simulink model "Lidar_System_July7_NoSerial"  (Simulink 7.3)
settings: Solver=FixedStepDiscrete  StartTime=0.0  StopTime=inf  FixedStep=0.1  MaxStep=0.2  RelTol=1e-3
libraries: dspmtrx3 x3, simulink x2, vipstatistics x2, dspstat3 x2, vipgeotforms x1
(part 1 of 2)
settings Model: Creator=gclayton  LastModifiedBy=wildcat
settings DebuggingCC: InheritedTsInSrcMsg=none
settings RTWCC: SystemTargetFile=rlnx.tlc  GenCodeOnly=on  TemplateMakefile=rlnx_ubuntu.tmf  Description=Linux Real-Time Target  ProcessScript=rlnx_make_rtw_hook
settings RTWCC: CustomInclude=|
  | /usr/local/include/opencv/
  | /usr/local/include/
settings CodeAppCC: GenerateComments=off  SimulinkBlockComments=off
settings STFCustomTargetCC: ModelReferenceCompliant=off  MatFileLogging=on  SystemTargetFile=rlnx.tlc
settings GRTTargetCC: ModelReferenceCompliant=off  ParMdlRefBuildCompliant=off  CompOptLevelCompliant=off
settings CustomProperty: DataType=string  Value="-lm -ldl /usr/local/lib/libopencv_highgui.so.2.4 /usr/local/lib/libopencv_core.so.2.4 /usr/local/lib/libopencv_imgproc.so.2.4  -lc_urg -lc_urg_connection -lc_urg_system -lphidget21"
settings EnumStrPairs: String=PC

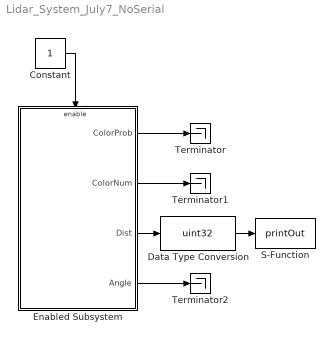
== system Lidar_System_July7_NoSerial ==
  Constant : Constant  OutDataType=fixdt(1, 16)  OutScaling=2^0
  Data Type Conversion : DataTypeConversion  OutDataTypeMode=uint32  OutDataType=fixdt(1, 16)  OutScaling=2^0  OutDataTypeStr=uint32
  Enabled Subsystem : Subsystem  TreatAsAtomicUnit=on
  S-Function : S-Function  FunctionName=printOut  EnableBusSupport=off
  Terminator : Terminator
  Terminator1 : Terminator
  Terminator2 : Terminator
  wires:
  Constant/1 -> Enabled Subsystem/Enable
  Enabled Subsystem/3(Dist) -> Data Type Conversion/1
  Data Type Conversion/1 -> S-Function/1
  Enabled Subsystem/1(ColorProb) -> Terminator/1
  Enabled Subsystem/2(ColorNum) -> Terminator1/1
  Enabled Subsystem/4(Angle) -> Terminator2/1

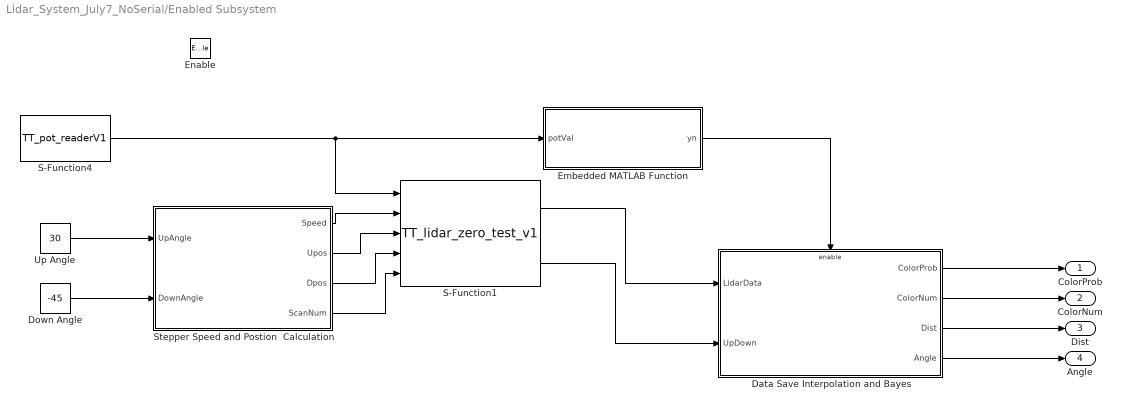
== system Lidar_System_July7_NoSerial/Enabled Subsystem ==
  Enable : EnablePort
  Data Save Interpolation and Bayes : Subsystem  TreatAsAtomicUnit=on
  Down Angle : Constant  Value=-45  OutDataType=fixdt(1, 16)  OutScaling=2^0
  Embedded MATLAB Function : Stateflow chart
  S-Function1 : S-Function  FunctionName=TT_lidar_zero_test_v1  EnableBusSupport=off
  S-Function4 : S-Function  FunctionName=TT_pot_readerV1  EnableBusSupport=off
  Stepper Speed and Postion  Calculation : Stateflow chart
  Up Angle : Constant  Value=30  OutDataType=fixdt(1, 16)  OutScaling=2^0
  ColorProb : Outport  OutDataType=fixdt(1, 16)  OutScaling=2^0
  ColorNum : Outport  Port=2  OutDataType=fixdt(1, 16)  OutScaling=2^0
  Dist : Outport  Port=3  OutDataType=fixdt(1, 16)  OutScaling=2^0
  Angle : Outport  Port=4  OutDataType=fixdt(1, 16)  OutScaling=2^0
  wires:
  S-Function4/1 -> S-Function1/1, Embedded MATLAB Function/1(potVal)
  Stepper Speed and Postion  Calculation/1(Speed) -> S-Function1/2
  Stepper Speed and Postion  Calculation/2(Upos) -> S-Function1/3
  Stepper Speed and Postion  Calculation/3(Dpos) -> S-Function1/4
  Stepper Speed and Postion  Calculation/4(ScanNum) -> S-Function1/5
  Embedded MATLAB Function/1(yn) -> Data Save Interpolation and Bayes/Enable
  S-Function1/1 -> Data Save Interpolation and Bayes/1(LidarData)
  S-Function1/2 -> Data Save Interpolation and Bayes/2(UpDown)
  Data Save Interpolation and Bayes/1(ColorProb) -> ColorProb/1
  Data Save Interpolation and Bayes/2(ColorNum) -> ColorNum/1
  Data Save Interpolation and Bayes/3(Dist) -> Dist/1
  Data Save Interpolation and Bayes/4(Angle) -> Angle/1
  Down Angle/1 -> Stepper Speed and Postion  Calculation/2(DownAngle)
  Up Angle/1 -> Stepper Speed and Postion  Calculation/1(UpAngle)

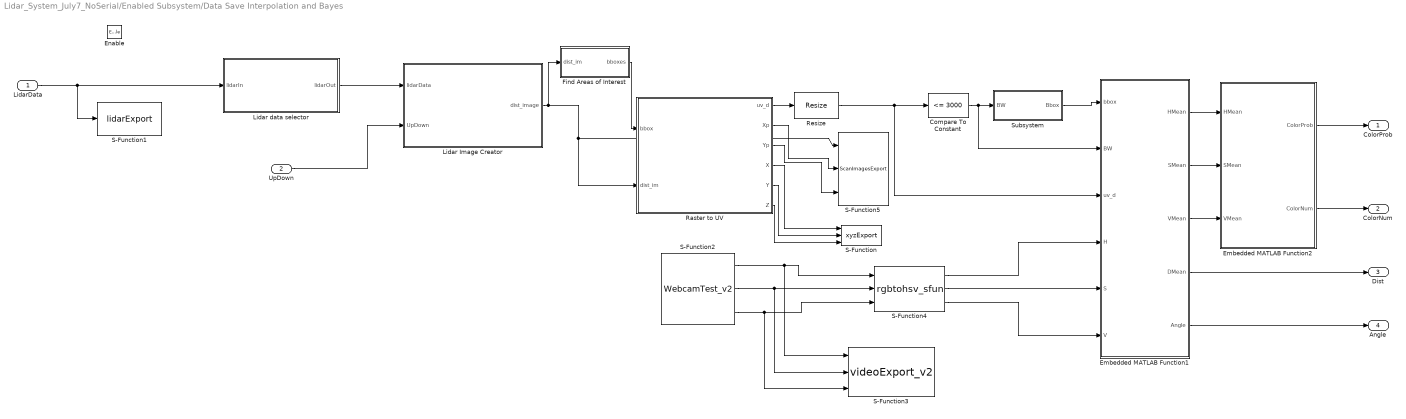
== system Lidar_System_July7_NoSerial/Enabled Subsystem/Data Save Interpolation and Bayes ==
  LidarData : Inport  OutDataType=fixdt(1, 16)  OutScaling=2^0
  UpDown : Inport  Port=2  OutDataType=fixdt(1, 16)  OutScaling=2^0
  Enable : EnablePort
  Compare To Constant : simulink/Logic and Bit Operations/Compare To Constant  SystemSampleTime=-1  relop=<=  const=3000  LogicOutDataTypeMode=boolean  ZeroCross=off
  Embedded MATLAB Function1 : Stateflow chart
  Embedded MATLAB Function2 : Stateflow chart
  Find Areas of Interest : Subsystem
  Lidar Image Creator : Stateflow chart
  Lidar data selector : Stateflow chart
  Raster to UV : Stateflow chart
  Resize : vipgeotforms/Resize  DialogController=vipDDGCreate  DialogControllerArgs=DataTag2  specify=Number of output rows and columns  rfactor=[200 150]  outCols=25  outRows=25  outRowsCols=[480 640]  interp_method=Bilinear  antialias=on  useROI=off  roiFlag=off  prodOutputMode=Binary point scaling  prodOutputWordLength=32  prodOutputFracLength=10  roundingMode=Nearest  overflowMode=on
  S-Function : S-Function  FunctionName=xyzExport  EnableBusSupport=off
  S-Function1 : S-Function  FunctionName=lidarExport  EnableBusSupport=off
  S-Function2 : S-Function  FunctionName=WebcamTest_v2  EnableBusSupport=off
  S-Function3 : S-Function  FunctionName=videoExport_v2  EnableBusSupport=off
  S-Function4 : S-Function  FunctionName=rgbtohsv_sfun  EnableBusSupport=off
  S-Function5 : S-Function  FunctionName=ScanImagesExport  EnableBusSupport=off
  Subsystem : Subsystem
  ColorProb : Outport  OutDataType=fixdt(1, 16)  OutScaling=2^0
  ColorNum : Outport  Port=2  OutDataType=fixdt(1, 16)  OutScaling=2^0
  Dist : Outport  Port=3  OutDataType=fixdt(1, 16)  OutScaling=2^0
  Angle : Outport  Port=4  OutDataType=fixdt(1, 16)  OutScaling=2^0
  wires:
  Lidar data selector/1(lidarOut) -> Lidar Image Creator/1(lidarData)
  UpDown/1 -> Lidar Image Creator/2(UpDown)
  Lidar Image Creator/1(dist_image) -> Find Areas of Interest/1(dist_im), Raster to UV/2(dist_im), S-Function5/1
  Find Areas of Interest/1(bboxes) -> Raster to UV/1(bbox)
  Compare To Constant/1 -> Subsystem/1(BW), Embedded MATLAB Function1/2(BW)
  Subsystem/1(Bbox) -> Embedded MATLAB Function1/1(bbox)
  Embedded MATLAB Function1/3(VMean) -> Embedded MATLAB Function2/3(VMean)
  Embedded MATLAB Function1/2(SMean) -> Embedded MATLAB Function2/2(SMean)
  Embedded MATLAB Function1/1(HMean) -> Embedded MATLAB Function2/1(HMean)
  Raster to UV/1(uv_d) -> Resize/1
  Embedded MATLAB Function2/1(ColorProb) -> ColorProb/1
  Embedded MATLAB Function2/2(ColorNum) -> ColorNum/1
  Embedded MATLAB Function1/5(Angle) -> Angle/1
  Embedded MATLAB Function1/4(DMean) -> Dist/1
  S-Function2/1 -> S-Function4/1, S-Function3/1
  S-Function2/2 -> S-Function4/2, S-Function3/2
  S-Function2/3 -> S-Function4/3, S-Function3/3
  S-Function4/1 -> Embedded MATLAB Function1/4(H)
  S-Function4/2 -> Embedded MATLAB Function1/5(S)
  S-Function4/3 -> Embedded MATLAB Function1/6(V)
  LidarData/1 -> Lidar data selector/1(lidarIn), S-Function1/1
  Resize/1 -> Compare To Constant/1, Embedded MATLAB Function1/3(uv_d)
  Raster to UV/2(Xp) -> S-Function5/2
  Raster to UV/4(X) -> S-Function/1
  Raster to UV/5(Y) -> S-Function/2
  Raster to UV/6(Z) -> S-Function/3
  Raster to UV/3(Yp) -> S-Function5/3

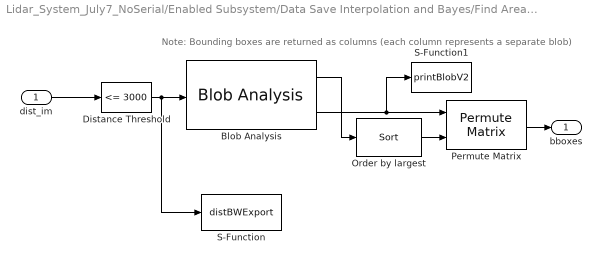
== system Lidar_System_July7_NoSerial/Enabled Subsystem/Data Save Interpolation and Bayes/Find Areas of Interest ==
  note: Note: Bounding boxes are returned as columns (each column represents a separate blob)
  dist_im : Inport  OutDataType=fixdt(1, 16)  OutScaling=2^0
  Blob Analysis : vipstatistics/Blob Analysis  DialogController=vipDDGCreate  DialogControllerArgs=DataTag0  area=on  centroid=off  bBox=on  majorAxis=off  minorAxis=off  angle=off  eccentricity=off  equivDiameterSq=off  extent=off  perimeter=off  maxBlobs=8  warnIfNumBlobsExceeded=on  isCount=off  useMinArea=on  minArea=30  useMaxArea=off  maxArea=intmax('uint32')  excludeBorderBlob=off  outDT=double  isOutVarDim=off  isFill=on  fillValues=-1  conn=8  isLabel=off  outputMode=Binary point scaling  outputWordLength=32  outputFracLength=16  firstCoeffMode=Binary point scaling  firstCoeffWordLength=16  firstCoeffFracLength=14  secondCoeffMode=Binary point scaling  secondCoeffWordLength=32  secondCoeffFracLength=16  accumMode=Binary point scaling  accumWordLength=32  accumFracLength=0  prodOutputMode=Binary point scaling  prodOutputWordLength=32  prodOutputFracLength=16  roundingMode=Floor  overflowMode=off
  Distance Threshold : simulink/Logic and Bit Operations/Compare To Constant  SystemSampleTime=-1  relop=<=  const=3000  LogicOutDataTypeMode=boolean  ZeroCross=off
  Order by largest : dspstat3/Sort  DialogController=dspDDGCreate  DialogControllerArgs=DataTag1  otype=Index  dir=Descending  sortAlg=Quick sort  roundingMode=Floor  overflowMode=off
  Permute Matrix : dspmtrx3/Permute Matrix  mode=Columns  ZeroOneIdxMode=One-based  errmode=Clip index  checkDims=off
  S-Function : S-Function  FunctionName=distBWExport  EnableBusSupport=off
  S-Function1 : S-Function  FunctionName=printBlobV2  EnableBusSupport=off
  bboxes : Outport  OutDataType=fixdt(1, 16)  OutScaling=2^0
  wires:
  dist_im/1 -> Distance Threshold/1
  Distance Threshold/1 -> Blob Analysis/1, S-Function/1
  Blob Analysis/2 -> Permute Matrix/1, S-Function1/1
  Order by largest/1 -> Permute Matrix/2
  Blob Analysis/1 -> Order by largest/1
  Permute Matrix/1 -> bboxes/1

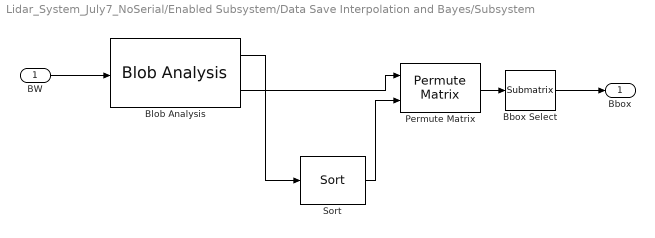
== system Lidar_System_July7_NoSerial/Enabled Subsystem/Data Save Interpolation and Bayes/Subsystem ==
  BW : Inport  OutDataType=fixdt(1, 16)  OutScaling=2^0
  Bbox Select : dspmtrx3/Submatrix  RowSpan=All rows  RowStartMode=First  RowStartIndex=1  RowEndMode=Last  RowEndIndex=1  ColSpan=One column  ColStartMode=First  ColStartIndex=1  ColEndMode=Last  ColEndIndex=1
  Blob Analysis : vipstatistics/Blob Analysis  DialogController=vipDDGCreate  DialogControllerArgs=DataTag3  area=on  centroid=off  bBox=on  majorAxis=off  minorAxis=off  angle=off  eccentricity=off  equivDiameterSq=off  extent=off  perimeter=off  maxBlobs=20  warnIfNumBlobsExceeded=on  isCount=off  useMinArea=on  minArea=20  useMaxArea=off  maxArea=intmax('uint32')  excludeBorderBlob=off  outDT=double  isOutVarDim=off  isFill=on  fillValues=-1  conn=8  isLabel=off  outputMode=Binary point scaling  outputWordLength=32  outputFracLength=16  firstCoeffMode=Binary point scaling  firstCoeffWordLength=16  firstCoeffFracLength=14  secondCoeffMode=Binary point scaling  secondCoeffWordLength=32  secondCoeffFracLength=16  accumMode=Binary point scaling  accumWordLength=32  accumFracLength=0  prodOutputMode=Binary point scaling  prodOutputWordLength=32  prodOutputFracLength=16  roundingMode=Floor  overflowMode=off
  Permute Matrix : dspmtrx3/Permute Matrix  mode=Columns  ZeroOneIdxMode=One-based  errmode=Clip index  checkDims=off
  Sort : dspstat3/Sort  DialogController=dspDDGCreate  DialogControllerArgs=DataTag4  otype=Index  dir=Descending  sortAlg=Quick sort  roundingMode=Floor  overflowMode=off
  Bbox : Outport  OutDataType=fixdt(1, 16)  OutScaling=2^0
  wires:
  BW/1 -> Blob Analysis/1
  Blob Analysis/1 -> Sort/1
  Sort/1 -> Permute Matrix/2
  Blob Analysis/2 -> Permute Matrix/1
  Permute Matrix/1 -> Bbox Select/1
  Bbox Select/1 -> Bbox/1

== matlab function Enabled Subsystem/Stepper Speed and Postion Calculation ==
  data: UpAngle input double; Speed output double; DownAngle input double; Upos output double; Dpos output double; ScanNum output double
function [Speed,Upos,Dpos,ScanNum] = stepper_calc(UpAngle,DownAngle)
% Last Edited by Anderson Lebbad on July 7, 2014
% edits were made to account for new calibration on gimbal

% This function inputs desired positive and negative scan angles
% and desired number of scans and outputs results positions for
% the stepper and the required speed of the stepper motor to properly
% move so the desired number of scans is obtained over the course of
% the motion of the stepper

% Scan Number requires no change
ScanNum = 65;
% Number of steps for 180 degree flip
stepRes = 3950;
% Parameter to account for slack in the gears with respect to steps
stepGive = 57;

% Transformation of angle to stepper position obtained from stepper calibration
% Output must be an integer
% 57 is added or subtracted due to wobble of gimbal system
Upos = round(UpAngle*stepRes/180)-stepGive;
Dpos = round(DownAngle*stepRes/180)+stepGive;

% Transformation of speed based 
% Output must be an interger
Speed = round(abs(UpAngle-DownAngle) * (1214/90));

== matlab function Enabled Subsystem/Embedded MATLAB Function ==
  data: potVal input double; yn output double
function yn = check_pot_val(potVal)
%#eml

% Pot value may initially be zero.
% Check for this and output a 1 or zero to 
% control whether the rest of model runs
if (potVal == 0)
    yn = 0;
else
    yn = 1;
end

== matlab function Enabled Subsystem/Data Save Interpolation and Bayes/Lidar data selector ==
  data: lidarIn input double; lidarOut output double
function lidarOut = data_selector(lidarIn)
% Lidar data is always input as a 1x70200 matrix.
% If Scan Number is less than 65 some of this data may be blank
% Select only the parts of the matrix where data has been collected

FullLength = 1080*65;
DataLength =  1080*65;
lidarOut = zeros(FullLength,1);

% ClosePts = (lidarIn < 3);
% lidarOut = (lidarIn + 30000*ClosePts)/10;

for i = 1:DataLength
    if (lidarIn(i,1) < 3)
        lidarIn(i,1) = 30000;
    end
    lidarOut(i,1) = lidarIn(i,1);
end

%lidarOut = lidarIn(1,1:DataLength);

== matlab function Enabled Subsystem/Data Save Interpolation and Bayes/Lidar Image Creator ==
  data: lidarData input double; dist_image output double; UpDown input double
function dist_image = scanImages(lidarData,UpDown)
%Written by Anderson Lebbad on July 5, 2014
%Last Edited:

%Converts the one dimensional array of lidarData and the scan settings into
%frames of distances and angles for each point

% Set output sizes
dist_image = zeros(65,540);

% To run through the middle half of the points horizonatal points, the
% first quarter must be skipped (of 1080)
scanOffset = 270-1;

% Loop through all points in output matrices
for j=1:540
    for i=1:65
        % Select the lidarData that will be used in analysis and format as
        % a frame
        dist_image(i,j) = lidarData(j+scanOffset+1080*(i-1));
    end
end

% Flip if up scan
if UpDown
    dist_image = flipud(dist_image);
end

dist_image = fliplr(dist_image);

end

== matlab function Enabled Subsystem/Data Save Interpolation and Bayes/Raster to UV ==
  data: bbox input double; uv_d output double; dist_im input double; Xp output double; Yp output double; X output double; Y output double; Z output double
function [uv_d,Xp,Yp,X,Y,Z] = fcn(bbox,dist_im)
% Written by Anderson Lebbad on July 3, 2014
% Last Edited:
%
% This function transforms the lidar raster image into u,v coordinates,
% with an xyz transformation and change of perspective from the lidar to
% the camera

%% Set Variables

% Find the number of valid bounding boxes
numBBox = 8 - sum(bbox(1,:) == -1);

beyondRange = 30000;
uv_d = beyondRange*ones(120,160);

% Initialize size of X,Y and Z matrices
X = zeros(size(dist_im));
Y = zeros(size(dist_im));
Z = zeros(size(dist_im));
Xc = zeros(size(dist_im));
Yc = zeros(size(dist_im));
Zc = zeros(size(dist_im));
Xn = zeros(size(dist_im));
Yn = zeros(size(dist_im));
Xp = zeros(size(dist_im));
Yp = zeros(size(dist_im));
r2 = zeros(size(dist_im));
r6 = zeros(size(dist_im));
Xd = zeros(size(dist_im));
Yd = zeros(size(dist_im));

% Scan angles vector
scanAngle = [2.74453024876108,2.74016692563110,2.73580360250111,2.73144027937113,2.72707695624114,2.72271363311115,2.71835030998117,2.71398698685118,2.70962366372120,2.70526034059121,2.70089701746123,2.69653369433124,2.69217037120125,2.68780704807127,2.68344372494128,2.67908040181130,2.67471707868131,2.67035375555132,2.66599043242134,2.66162710929135,2.65726378616137,2.65290046303138,2.64853713990140,2.64417381677141,2.63981049364142,2.63544717051144,2.63108384738145,2.62672052425147,2.62235720112148,2.61799387799149,2.61363055486151,2.60926723173152,2.60490390860154,2.60054058547155,2.59617726234157,2.59181393921158,2.58745061608159,2.58308729295161,2.57872396982162,2.57436064669164,2.56999732356165,2.56563400043166,2.56127067730168,2.55690735417169,2.55254403104171,2.54818070791172,2.54381738478174,2.53945406165175,2.53509073852176,2.53072741539178,2.52636409226179,2.52200076913181,2.51763744600182,2.51327412287183,2.50891079974185,2.50454747661186,2.50018415348188,2.49582083035189,2.49145750722191,2.48709418409192,2.48273086096193,2.47836753783195,2.47400421470196,2.46964089157198,2.46527756844199,2.46091424531200,2.45655092218202,2.45218759905203,2.44782427592205,2.44346095279206,2.43909762966208,2.43473430653209,2.43037098340210,2.42600766027212,2.42164433714213,2.41728101401215,2.41291769088216,2.40855436775217,2.40419104462219,2.39982772149220,2.39546439836222,2.39110107523223,2.38673775210225,2.38237442897226,2.37801110584227,2.37364778271229,2.36928445958230,2.36492113645232,2.36055781332233,2.35619449019235,2.35183116706236,2.34746784393237,2.34310452080239,2.33874119767240,2.33437787454242,2.33001455141243,2.32565122828244,2.32128790515246,2.31692458202247,2.31256125889249,2.30819793576250,2.30383461263252,2.29947128950253,2.29510796637254,2.29074464324256,2.28638132011257,2.28201799698259,2.27765467385260,2.27329135072261,2.26892802759263,2.26456470446264,2.26020138133266,2.25583805820267,2.25147473507269,2.24711141194270,2.24274808881271,2.23838476568273,2.23402144255274,2.22965811942276,2.22529479629277,2.22093147316278,2.21656815003280,2.21220482690281,2.20784150377283,2.20347818064284,2.19911485751286,2.19475153438287,2.19038821125288,2.18602488812290,2.18166156499291,2.17729824186293,2.17293491873294,2.16857159560295,2.16420827247297,2.15984494934298,2.15548162621300,2.15111830308301,2.14675497995303,2.14239165682304,2.13802833369305,2.13366501056307,2.12930168743308,2.12493836430310,2.12057504117311,2.11621171804312,2.11184839491314,2.10748507178315,2.10312174865317,2.09875842552318,2.09439510239320,2.09003177926321,2.08566845613322,2.08130513300324,2.07694180987325,2.07257848674327,2.06821516361328,2.06385184048329,2.05948851735331,2.05512519422332,2.05076187109334,2.04639854796335,2.04203522483337,2.03767190170338,2.03330857857339,2.02894525544341,2.02458193231342,2.02021860918344,2.01585528605345,2.01149196292347,2.00712863979348,2.00276531666349,1.99840199353351,1.99403867040352,1.98967534727354,1.98531202414355,1.98094870101356,1.97658537788358,1.97222205475359,1.96785873162361,1.96349540849362,1.95913208536364,1.95476876223365,1.95040543910366,1.94604211597368,1.94167879284369,1.93731546971371,1.93295214658372,1.92858882345373,1.92422550032375,1.91986217719376,1.91549885406378,1.91113553093379,1.90677220780381,1.90240888467382,1.89804556154383,1.89368223841385,1.88931891528386,1.88495559215388,1.88059226902389,1.87622894589390,1.87186562276392,1.86750229963393,1.86313897650395,1.85877565337396,1.85441233024398,1.85004900711399,1.84568568398400,1.84132236085402,1.83695903772403,1.83259571459405,1.82823239146406,1.82386906833407,1.81950574520409,1.81514242207410,1.81077909894412,1.80641577581413,1.80205245268415,1.79768912955416,1.79332580642417,1.78896248329419,1.78459916016420,1.78023583703422,1.77587251390423,1.77150919077424,1.76714586764426,1.76278254451427,1.75841922138429,1.75405589825430,1.74969257512432,1.74532925199433,1.74096592886434,1.73660260573436,1.73223928260437,1.72787595947439,1.72351263634440,1.71914931321441,1.71478599008443,1.71042266695444,1.70605934382446,1.70169602069447,1.69733269756449,1.69296937443450,1.68860605130451,1.68424272817453,1.67987940504454,1.67551608191456,1.67115275878457,1.66678943565458,1.66242611252460,1.65806278939461,1.65369946626463,1.64933614313464,1.64497282000466,1.64060949687467,1.63624617374468,1.63188285061470,1.62751952748471,1.62315620435473,1.61879288122474,1.61442955809475,1.61006623496477,1.60570291183478,1.60133958870480,1.59697626557481,1.59261294244483,1.58824961931484,1.58388629618485,1.57952297305487,1.57515964992488,1.57079632679490,1.56643300366491,1.56206968053493,1.55770635740494,1.55334303427495,1.54897971114497,1.54461638801498,1.54025306488500,1.53588974175501,1.53152641862502,1.52716309549504,1.52279977236505,1.51843644923507,1.51407312610508,1.50970980297510,1.50534647984511,1.50098315671512,1.49661983358514,1.49225651045515,1.48789318732517,1.48352986419518,1.47916654106519,1.47480321793521,1.47043989480522,1.46607657167524,1.46171324854525,1.45734992541527,1.45298660228528,1.44862327915529,1.44425995602531,1.43989663289532,1.43553330976534,1.43116998663535,1.42680666350536,1.42244334037538,1.41808001724539,1.41371669411541,1.40935337098542,1.40499004785544,1.40062672472545,1.39626340159546,1.39190007846548,1.38753675533549,1.38317343220551,1.37881010907552,1.37444678594553,1.37008346281555,1.36572013968556,1.36135681655558,1.35699349342559,1.35263017029561,1.34826684716562,1.34390352403563,1.33954020090565,1.33517687777566,1.33081355464568,1.32645023151569,1.32208690838570,1.31772358525572,1.31336026212573,1.30899693899575,1.30463361586576,1.30027029273578,1.29590696960579,1.29154364647580,1.28718032334582,1.28281700021583,1.27845367708585,1.27409035395586,1.26972703082587,1.26536370769589,1.26100038456590,1.25663706143592,1.25227373830593,1.24791041517595,1.24354709204596,1.23918376891597,1.23482044578599,1.23045712265600,1.22609379952602,1.22173047639603,1.21736715326604,1.21300383013606,1.20864050700607,1.20427718387609,1.19991386074610,1.19555053761612,1.19118721448613,1.18682389135614,1.18246056822616,1.17809724509617,1.17373392196619,1.16937059883620,1.16500727570621,1.16064395257623,1.15628062944624,1.15191730631626,1.14755398318627,1.14319066005629,1.13882733692630,1.13446401379631,1.13010069066633,1.12573736753634,1.12137404440636,1.11701072127637,1.11264739814639,1.10828407501640,1.10392075188641,1.09955742875643,1.09519410562644,1.09083078249646,1.08646745936647,1.08210413623648,1.07774081310650,1.07337748997651,1.06901416684653,1.06465084371654,1.06028752058656,1.05592419745657,1.05156087432658,1.04719755119660,1.04283422806661,1.03847090493663,1.03410758180664,1.02974425867665,1.02538093554667,1.02101761241668,1.01665428928670,1.01229096615671,1.00792764302673,1.00356431989674,0.999200996766754,0.994837673636768,0.990474350506782,0.986111027376796,0.981747704246810,0.977384381116825,0.973021057986839,0.968657734856853,0.964294411726867,0.959931088596881,0.955567765466896,0.951204442336910,0.946841119206924,0.942477796076938,0.938114472946952,0.933751149816966,0.929387826686981,0.925024503556995,0.920661180427009,0.916297857297023,0.911934534167037,0.907571211037051,0.903207887907065,0.898844564777080,0.894481241647094,0.890117918517108,0.885754595387122,0.881391272257136,0.877027949127151,0.872664625997165,0.868301302867179,0.863937979737193,0.859574656607207,0.855211333477221,0.850848010347236,0.846484687217250,0.842121364087264,0.837758040957278,0.833394717827292,0.829031394697307,0.824668071567321,0.820304748437335,0.815941425307349,0.811578102177363,0.807214779047377,0.802851455917392,0.798488132787406,0.794124809657420,0.789761486527434,0.785398163397448,0.781034840267463,0.776671517137477,0.772308194007491,0.767944870877505,0.763581547747519,0.759218224617533,0.754854901487548,0.750491578357562,0.746128255227576,0.741764932097590,0.737401608967604,0.733038285837618,0.728674962707633,0.724311639577647,0.719948316447661,0.715584993317675,0.711221670187689,0.706858347057704,0.702495023927718,0.698131700797732,0.693768377667746,0.689405054537760,0.685041731407774,0.680678408277789,0.676315085147803,0.671951762017817,0.667588438887831,0.663225115757845,0.658861792627859,0.654498469497874,0.650135146367888,0.645771823237902,0.641408500107916,0.637045176977930,0.632681853847944,0.628318530717959,0.623955207587973,0.619591884457987,0.615228561328001,0.610865238198015,0.606501915068030,0.602138591938044,0.597775268808058,0.593411945678072,0.589048622548086,0.584685299418100,0.580321976288115,0.575958653158129,0.571595330028143,0.567232006898157,0.562868683768171,0.558505360638186,0.554142037508200,0.549778714378214,0.545415391248228,0.541052068118242,0.536688744988256,0.532325421858271,0.527962098728285,0.523598775598299,0.519235452468313,0.514872129338327,0.510508806208341,0.506145483078356,0.501782159948370,0.497418836818384,0.493055513688398,0.488692190558412,0.484328867428426,0.479965544298441,0.475602221168455,0.471238898038469,0.466875574908483,0.462512251778497,0.458148928648512,0.453785605518526,0.449422282388540,0.445058959258554,0.440695636128568,0.436332312998582,0.431968989868597,0.427605666738611,0.423242343608625,0.418879020478639,0.414515697348653,0.410152374218667,0.405789051088682,0.401425727958696,0.397062404828710,0.392699081698724];
% Gimbal angle vector
gimbalAngle = [0.503460361152210,0.483321946706122,0.463183532260034,0.443045117813945,0.422906703367857,0.402768288921768,0.382629874475680,0.362491460029592,0.342353045583503,0.322214631137415,0.302076216691326,0.281937802245238,0.261799387799149,0.241660973353061,0.221522558906973,0.201384144460884,0.181245730014796,0.161107315568707,0.140968901122619,0.120830486676531,0.100692072230442,0.0805536577843537,0.0604152433382652,0.0402768288921768,0.0201384144460884,0,-0.0201384144460884,-0.0402768288921768,-0.0604152433382652,-0.0805536577843536,-0.100692072230442,-0.120830486676530,-0.140968901122619,-0.161107315568707,-0.181245730014796,-0.201384144460884,-0.221522558906973,-0.241660973353061,-0.261799387799149,-0.281937802245238,-0.302076216691326,-0.322214631137415,-0.342353045583503,-0.362491460029592,-0.382629874475680,-0.402768288921768,-0.422906703367857,-0.443045117813945,-0.463183532260034,-0.483321946706122,-0.503460361152210,-0.523598775598299,-0.543737190044387,-0.563875604490476,-0.584014018936564,-0.604152433382653,-0.624290847828741,-0.644429262274829,-0.664567676720918,-0.684706091167006,-0.704844505613095,-0.724982920059183,-0.745121334505272,-0.765259748951360,-0.785398163397448];

% Height of the lidar on the gimbal
h = 36.3;

% Translation vector (in milliimeters)
t = [24; -113; 38];

% Rotation angles
phi = (-90+6)*pi/180;
theta = 0*pi/180;

% Rotation about the x-axis
Rx = [1 0 0; 0 cos(phi) sin(phi); 0 -sin(phi) cos(phi)];
% Followed by rotation about the y-axis
R = [cos(theta) 0 -sin(theta); 0 1 0; sin(theta) 0 cos(theta)]*Rx;

% Transformation matrix
T = [R t];

% Radial Distortions
RadDist = [0.069102182282360,-0.154608606024690,0.020241053576861];

% Intrinsic Matrix
K = [5.548581600685270e+02,0,0;0,5.523116000564020e+02,0;3.135858904821101e+02,2.190392333699872e+02,1];
KK = K';

% Iterate filling points into XYZ matrices for each valid bbox
for i = 1:numBBox
       
    % Find region to fill
    minX = bbox(2,i) + 1;
    maxX = minX + bbox(4,i) - 1;
    minY = bbox(1,i) + 1;
    maxY = minY + bbox(3,i) - 1;
    
    % Loop for each pixel in the bounding box
    for j = minX:maxX
        for k = minY:maxY  
            % Convert to XYZ
            X(k,j) = dist_im(k,j).*cos(scanAngle(j));
            Y(k,j) = dist_im(k,j).*sin(scanAngle(j)).*cos(gimbalAngle(i))-h.*sin(gimbalAngle(i));
            Z(k,j) = dist_im(k,j).*sin(scanAngle(j)).*sin(gimbalAngle(i))+h.*cos(gimbalAngle(i));
            
            % Transformation to camera coordinate frame
            Xc(k,j) = T(1,1)*X(k,j)+T(1,2)*Y(k,j)+T(1,3)*Z(k,j)+T(1,4);
            Yc(k,j) = T(2,1)*X(k,j)+T(2,2)*Y(k,j)+T(2,3)*Z(k,j)+T(2,4);
            Zc(k,j) = T(3,1)*X(k,j)+T(3,2)*Y(k,j)+T(3,3)*Z(k,j)+T(3,4);
            
            % Normalize Coordinates
            Xn(k,j) = Xc(k,j)./Zc(k,j);
            Yn(k,j) = Yc(k,j)./Zc(k,j);
            
            % Radial Vectors
            r2(k,j) = Xn(k,j).^2+Yn(k,j).^2;
            r6(k,j) = r2(k,j).^3;
            
            % Distorted Coodinates
            Xd(k,j) = Xn(k,j).*(1+RadDist(1).*r2(k,j)+RadDist(3).*r6(k,j));
            Yd(k,j) = Yn(k,j).*(1+RadDist(1).*r2(k,j)+RadDist(3).*r6(k,j));
            
            % Pixel Coordinates
            Xp(k,j) = KK(1,1)*Xd(k,j)+KK(1,2)*Yd(k,j)+KK(1,3);
            Yp(k,j) = KK(2,1)*Xd(k,j)+KK(2,2)*Yd(k,j)+KK(2,3);
        end
    end
end

% Depth frame, same aspect ratio as image frame, quarter width and height
for i2 = 1:160
    for j2 = 1:120
        % Estimated Closest points
        xCenter = int32(146+i2*1.55);
        yCenter = int32(j2/1.8462);
        
        % Evaluate once for reference
        l1norm = abs(Xp(yCenter,xCenter)-i2*4-2)+abs(Yp(yCenter,xCenter)-j2*4-2);
        uv_d(j2,i2) = dist_im(yCenter,xCenter);
        
        % Loop over a region of interest near estimated point
        for m = xCenter-3:xCenter+3
            for n = yCenter-3:yCenter+3
                % Check to see if dist coordinate is valid (only need to check y)
                if (n > 0) && (n < 65)
                    % Check if l1norm is smaller than previous smallest
                    if (abs(Xp(n,m)-i2*4-2)+abs(Yp(n,m)-j2*4-2)) < l1norm
                        l1norm = abs(Xp(n,m)-i2*4-2)+abs(Yp(n,m)-j2*4-2);
                        uv_d(j2,i2) = dist_im(n,m);
                    end
                end
            end
        end
    end
end

end

== matlab function Enabled Subsystem/Data Save Interpolation and Bayes/Embedded MATLAB Function1 ==
  data: bbox input double; HMean output double; BW input double; uv_d input double; H input double; S input double; V input double; SMean output double; VMean output double; DMean output double; Angle output double
function [HMean, SMean, VMean, DMean, Angle] = bbox_hist(bbox, BW, uv_d, H, S, V)
%This function creates a histogram of the color region of a detected object
%identified in a binary image within a bounding box

%Initialize variables
pixels = 0;
DRunAve = 0;
HRunAve = 0;
SRunAve = 0;
VRunAve = 0;
CDist = 0;
FoV = 62;

%Parse bbox data
left = bbox(2) + 1;
right = left + bbox(4) - 1;
bottom = bbox(1) + 1;
top = bottom + bbox(3) - 1;
Angle = int32((left + bbox(4)/2-320)/320*FoV/2);

%Check to see if valid bbox is found
if left~=-1
    %Scan the detected region of the binary image and generate histograms
    for j=left:right
        for i=bottom:top
            if BW(i,j) == 1
                pixels = pixels + 1;
                DRunAve = ((pixels-1)/pixels)*DRunAve + (1/pixels)*double(uv_d(i,j));
                HRunAve = ((pixels-1)/pixels)*HRunAve + (1/pixels)*double(H(i,j));
                SRunAve = ((pixels-1)/pixels)*SRunAve + (1/pixels)*double(S(i,j));
                VRunAve = ((pixels-1)/pixels)*VRunAve + (1/pixels)*double(V(i,j));
            end
        end
    end
    %CDist = uv_d(left,right);
end

%Means must be integers to use in Bayes Filter
DMean = int32(DRunAve/10);
%DMean = int32(CDist);
HMean = uint8(HRunAve);
SMean = uint8(SRunAve);
VMean = uint8(VRunAve);

end
